simulink model "X_to_ADD_fix"  (Simulink 7.0)
settings: Solver=FixedStepDiscrete  SolverMode=SingleTasking  StartTime=0.0  StopTime=1100  FixedStep=Ts  RelTol=1e-3
values from neighbouring files (symbols this model uses):
  Ts = 1    [x_to_add_fix_init.m]
  x_data_nb = 16    [x_to_add_fix_init.m]
  x_range_nb = 16    [x_to_add_fix_init.m]
undefined symbols (not defined in the file or in its folder): xlipgetpartsetting
libraries: xbsIndex_r4 x55
settings Model: Creator=jboulet  LastModifiedBy=jboulet

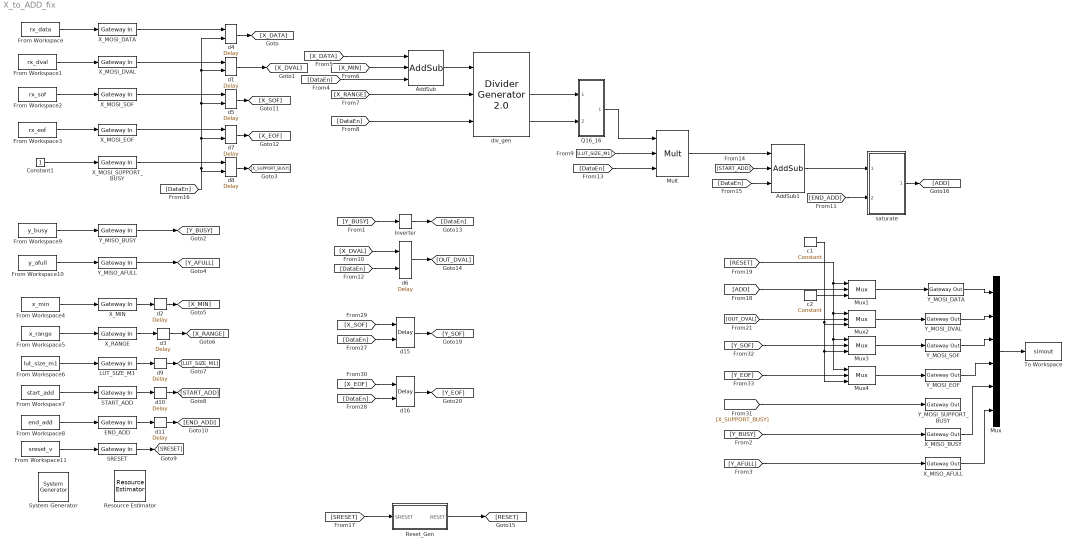
== system X_to_ADD_fix ==
  " System Generator" : xbsIndex_r4/ System Generator  Tag=genX  SystemSampleTime=-1  xilinxfamily=virtex4  part=xc4vfx100  speed=-10  package=ff1517  synthesis_tool=XST  clock_wrapper=Expose Clock Ports  directory=./ngc_netlist  testbench=off  simulink_period=1  sysclk_period=7.5  dcm_input_clock_period=100  incr_netlist=off  trim_vbits=Everywhere in SubSystem  dbl_ovrd=According to Block Masks  core_generation=According to Block Masks  run_coregen=off  deprecated_control=off  eval_field=0  block_type=sysgen
      settings: block_version=10.1.3
  AddSub : xbsIndex_r4/AddSub  mode=Subtraction  use_carryin=off  use_carryout=off  en=on  latency=1  precision=User Defined  arith_type=Unsigned  n_bits=16  bin_pt=0  quantization=Truncate  overflow=Saturate  dbl_ovrd=off  use_behavioral_HDL=off  pipelined=off  use_rpm=off  hw_selection=Fabric  block_type=addsub
      settings: xl_area=[8 16 0 16 0 0 0]  block_version=10.1.3
  AddSub1 : xbsIndex_r4/AddSub  mode=Addition  use_carryin=off  use_carryout=off  en=on  latency=1  precision=User Defined  arith_type=Unsigned  n_bits=end_add_nb  bin_pt=0  quantization=Truncate  overflow=Wrap  dbl_ovrd=off  use_behavioral_HDL=off  pipelined=off  use_rpm=on  hw_selection=Fabric  block_type=addsub
      settings: xl_area=[5 10 0 10 0 0 0]  block_version=10.1.3
  Constant1 : Constant
  END_ADD : xbsIndex_r4/Gateway In  arith_type=Unsigned  n_bits=end_add_nb  bin_pt=0  quantization=Truncate  overflow=Wrap  period=Ts  dbl_ovrd=off  timing_constraint=None  locs_specified=off  LOCs={}  block_type=gatewayin
      settings: infoedit="Gateway in block.  Converts inputs of type Simulink integer, double and fixed point to  Xilinx fixed point type.<P><P>Hardware notes:  In hardware these blocks become top level input ports."  xl_area=[0 0 0 0 10 0 0]  block_version=10.1.3
  From Workspace : FromWorkspace  VariableName=rx_data  SampleTime=Ts  Interpolate=off  OutputAfterFinalValue=Holding final value
  From Workspace1 : FromWorkspace  VariableName=rx_dval  SampleTime=Ts  Interpolate=off  OutputAfterFinalValue=Setting to zero
  From Workspace10 : FromWorkspace  VariableName=y_afull  SampleTime=Ts  Interpolate=off  OutputAfterFinalValue=Holding final value
  From Workspace11 : FromWorkspace  VariableName=sreset_v  SampleTime=Ts  Interpolate=off  OutputAfterFinalValue=Holding final value
  From Workspace2 : FromWorkspace  VariableName=rx_sof  SampleTime=Ts  Interpolate=off  OutputAfterFinalValue=Holding final value
  From Workspace3 : FromWorkspace  VariableName=rx_eof  SampleTime=Ts  Interpolate=off  OutputAfterFinalValue=Holding final value
  From Workspace4 : FromWorkspace  VariableName=x_min  SampleTime=Ts  Interpolate=off  OutputAfterFinalValue=Holding final value
  From Workspace5 : FromWorkspace  VariableName=x_range  SampleTime=Ts  Interpolate=off  OutputAfterFinalValue=Holding final value
  From Workspace6 : FromWorkspace  VariableName=lut_size_m1  SampleTime=Ts  Interpolate=off  OutputAfterFinalValue=Holding final value
  From Workspace7 : FromWorkspace  VariableName=start_add  SampleTime=Ts  Interpolate=off  OutputAfterFinalValue=Holding final value
  From Workspace8 : FromWorkspace  VariableName=end_add  SampleTime=Ts  Interpolate=off  OutputAfterFinalValue=Holding final value
  From Workspace9 : FromWorkspace  VariableName=y_busy  SampleTime=Ts  Interpolate=off  OutputAfterFinalValue=Holding final value
  Inverter : xbsIndex_r4/Inverter  en=off  latency=0  dbl_ovrd=off  block_type=inv
      settings: xl_area=[0 0 0 0 0 0 0]
  LUT_SIZE_M1 : xbsIndex_r4/Gateway In  arith_type=Unsigned  n_bits=lut_size_m1_nb  bin_pt=0  quantization=Truncate  overflow=Wrap  period=Ts  dbl_ovrd=off  timing_constraint=None  locs_specified=off  LOCs={}  block_type=gatewayin
      settings: infoedit="Gateway in block.  Converts inputs of type Simulink integer, double and fixed point to  Xilinx fixed point type.<P><P>Hardware notes:  In hardware these blocks become top level input ports."  xl_area=[0 0 0 0 10 0 0]  block_version=10.1.3
  Mult : xbsIndex_r4/Mult  precision=User Defined  arith_type=Unsigned  n_bits=end_add_nb  bin_pt=0  quantization=Truncate  overflow=Wrap  en=on  latency=3  dbl_ovrd=off  use_behavioral_HDL=off  use_embedded=off  opt=Speed  optimum_pipeline=off  pipeline=on  use_rpm=on  placement_style=Triangular  block_type=mult
      settings: infoedit=Hardware notes: To use the internal pipeline stage of the dedicated multiplier you must select 'Pipeline for maximum performance'.  xl_area=[119 209 0 198 0 0 0]  block_version=10.1.3
  Mux : Mux  Inputs=6
  Mux{1..4} (4 alike) : xbsIndex_r4/Mux  inputs=2  en=off  latency=0  precision=Full  arith_type=Unsigned  n_bits=16  bin_pt=14  quantization=Truncate  overflow=Wrap  dbl_ovrd=off  block_type=mux
  Q16_16 : Subsystem
  Reset_Gen : Subsystem
  Resource Estimator : xbsIndex_r4/Resource Estimator  Tag=resEstTag  Slices=88  FFs=61  BRAMs=1  LUTs=84  IOBs=48  EBMs=0  TBUFs=0  xl_use_estimator_area=off  est_options=Estimate  xl_estimator_area=[188 318 0 246 137 0 0]  block_type=resource_estimator
      settings: AttributesFormatString=Resource\nEstimator  block_version=10.1.3
  SRESET : xbsIndex_r4/Gateway In  arith_type=Boolean  n_bits=8  bin_pt=0  quantization="Round  (unbiased: +/- Inf)"  overflow=Wrap  period=1  dbl_ovrd=off  timing_constraint=None  locs_specified=off  LOCs={}  block_type=gatewayin
      settings: infoedit="Gateway in block.  Converts inputs of type Simulink integer, double and fixed point to  Xilinx fixed point type.<P><P>Hardware notes:  In hardware these blocks become top level input ports."  xl_area=[0 0 0 0 1 0 0]  block_version=10.1.3
  START_ADD : xbsIndex_r4/Gateway In  arith_type=Unsigned  n_bits=start_add_nb  bin_pt=0  quantization=Truncate  overflow=Wrap  period=Ts  dbl_ovrd=off  timing_constraint=None  locs_specified=off  LOCs={}  block_type=gatewayin
      settings: infoedit="Gateway in block.  Converts inputs of type Simulink integer, double and fixed point to  Xilinx fixed point type.<P><P>Hardware notes:  In hardware these blocks become top level input ports."  xl_area=[0 0 0 0 10 0 0]  block_version=10.1.3
  To Workspace : ToWorkspace  VariableName=simout  SampleTime=-1  SaveFormat=Structure
  X_MIN : xbsIndex_r4/Gateway In  arith_type=Unsigned  n_bits=x_min_nb  bin_pt=0  quantization=Truncate  overflow=Wrap  period=Ts  dbl_ovrd=off  timing_constraint=None  locs_specified=off  LOCs={}  block_type=gatewayin
      settings: infoedit="Gateway in block.  Converts inputs of type Simulink integer, double and fixed point to  Xilinx fixed point type.<P><P>Hardware notes:  In hardware these blocks become top level input ports."  xl_area=[0 0 0 0 16 0 0]  block_version=10.1.3
  X_MISO_AFULL : xbsIndex_r4/Gateway Out  hdl_port=on  timing_constraint=None  locs_specified=off  LOCs={}  block_type=gatewayout
      settings: infoedit="Gateway out block.  Converts Xilinx fixed point inputs into ouputs of type Simulink integer, double, or fixed point.<P><P>Hardware notes:  In hardware these blocks become top level output ports or are discarded, depending on how they are configured."  xl_area=[0 0 0 0 1 0 0]  block_version=10.1.3
  X_MISO_BUSY : xbsIndex_r4/Gateway Out  hdl_port=on  timing_constraint=None  locs_specified=off  LOCs={}  block_type=gatewayout
      settings: infoedit="Gateway out block.  Converts Xilinx fixed point inputs into ouputs of type Simulink integer, double, or fixed point.<P><P>Hardware notes:  In hardware these blocks become top level output ports or are discarded, depending on how they are configured."  xl_area=[0 0 0 0 1 0 0]  block_version=10.1.3
  X_MOSI_DATA : xbsIndex_r4/Gateway In  arith_type=Unsigned  n_bits=x_data_nb  bin_pt=0  quantization=Truncate  overflow=Wrap  period=Ts  dbl_ovrd=off  timing_constraint=None  locs_specified=off  LOCs={}  block_type=gatewayin
      settings: infoedit="Gateway in block.  Converts inputs of type Simulink integer, double and fixed point to  Xilinx fixed point type.<P><P>Hardware notes:  In hardware these blocks become top level input ports."  xl_area=[0 0 0 0 16 0 0]  block_version=10.1.3
  X_MOSI_DVAL : xbsIndex_r4/Gateway In  arith_type=Boolean  n_bits=8  bin_pt=0  quantization="Round  (unbiased: +/- Inf)"  overflow=Wrap  period=1  dbl_ovrd=off  timing_constraint=None  locs_specified=off  LOCs={}  block_type=gatewayin
      settings: infoedit="Gateway in block.  Converts inputs of type Simulink integer, double and fixed point to  Xilinx fixed point type.<P><P>Hardware notes:  In hardware these blocks become top level input ports."  xl_area=[0 0 0 0 1 0 0]  block_version=10.1.3
  X_MOSI_EOF : xbsIndex_r4/Gateway In  arith_type=Boolean  n_bits=8  bin_pt=0  quantization="Round  (unbiased: +/- Inf)"  overflow=Wrap  period=1  dbl_ovrd=off  timing_constraint=None  locs_specified=off  LOCs={}  block_type=gatewayin
      settings: infoedit="Gateway in block.  Converts inputs of type Simulink integer, double and fixed point to  Xilinx fixed point type.<P><P>Hardware notes:  In hardware these blocks become top level input ports."  xl_area=[0 0 0 0 1 0 0]  block_version=10.1.3
  X_MOSI_SOF : xbsIndex_r4/Gateway In  arith_type=Boolean  n_bits=8  bin_pt=0  quantization="Round  (unbiased: +/- Inf)"  overflow=Wrap  period=1  dbl_ovrd=off  timing_constraint=None  locs_specified=off  LOCs={}  block_type=gatewayin
      settings: infoedit="Gateway in block.  Converts inputs of type Simulink integer, double and fixed point to  Xilinx fixed point type.<P><P>Hardware notes:  In hardware these blocks become top level input ports."  xl_area=[0 0 0 0 1 0 0]  block_version=10.1.3
  X_MOSI_SUPPORT_BUSY : xbsIndex_r4/Gateway In  arith_type=Boolean  n_bits=8  bin_pt=0  quantization="Round  (unbiased: +/- Inf)"  overflow=Wrap  period=1  dbl_ovrd=off  timing_constraint=None  locs_specified=off  LOCs={}  block_type=gatewayin
      settings: infoedit="Gateway in block.  Converts inputs of type Simulink integer, double and fixed point to  Xilinx fixed point type.<P><P>Hardware notes:  In hardware these blocks become top level input ports."  xl_area=[0 0 0 0 1 0 0]  block_version=10.1.3
  X_RANGE : xbsIndex_r4/Gateway In  arith_type=Unsigned  n_bits=x_range_nb  bin_pt=0  quantization=Truncate  overflow=Wrap  period=Ts  dbl_ovrd=off  timing_constraint=None  locs_specified=off  LOCs={}  block_type=gatewayin
      settings: infoedit="Gateway in block.  Converts inputs of type Simulink integer, double and fixed point to  Xilinx fixed point type.<P><P>Hardware notes:  In hardware these blocks become top level input ports."  xl_area=[0 0 0 0 16 0 0]  block_version=10.1.3
  Y_MISO_AFULL : xbsIndex_r4/Gateway In  arith_type=Boolean  n_bits=8  bin_pt=0  quantization="Round  (unbiased: +/- Inf)"  overflow=Wrap  period=1  dbl_ovrd=off  timing_constraint=None  locs_specified=off  LOCs={}  block_type=gatewayin
      settings: infoedit="Gateway in block.  Converts inputs of type Simulink integer, double and fixed point to  Xilinx fixed point type.<P><P>Hardware notes:  In hardware these blocks become top level input ports."  xl_area=[0 0 0 0 1 0 0]  block_version=10.1.3
  Y_MISO_BUSY : xbsIndex_r4/Gateway In  arith_type=Boolean  n_bits=8  bin_pt=0  quantization="Round  (unbiased: +/- Inf)"  overflow=Wrap  period=1  dbl_ovrd=off  timing_constraint=None  locs_specified=off  LOCs={}  block_type=gatewayin
      settings: infoedit="Gateway in block.  Converts inputs of type Simulink integer, double and fixed point to  Xilinx fixed point type.<P><P>Hardware notes:  In hardware these blocks become top level input ports."  xl_area=[0 0 0 0 1 0 0]  block_version=10.1.3
  Y_MOSI_DATA : xbsIndex_r4/Gateway Out  hdl_port=on  timing_constraint=None  locs_specified=off  LOCs={}  block_type=gatewayout
      settings: infoedit="Gateway out block.  Converts Xilinx fixed point inputs into ouputs of type Simulink integer, double, or fixed point.<P><P>Hardware notes:  In hardware these blocks become top level output ports or are discarded, depending on how they are configured."  xl_area=[0 0 0 0 10 0 0]  block_version=10.1.3
  Y_MOSI_DVAL : xbsIndex_r4/Gateway Out  hdl_port=on  timing_constraint=None  locs_specified=off  LOCs={}  block_type=gatewayout
      settings: infoedit="Gateway out block.  Converts Xilinx fixed point inputs into ouputs of type Simulink integer, double, or fixed point.<P><P>Hardware notes:  In hardware these blocks become top level output ports or are discarded, depending on how they are configured."  xl_area=[0 0 0 0 10 0 0]  block_version=10.1.3
  Y_MOSI_EOF : xbsIndex_r4/Gateway Out  hdl_port=on  timing_constraint=None  locs_specified=off  LOCs={}  block_type=gatewayout
      settings: infoedit="Gateway out block.  Converts Xilinx fixed point inputs into ouputs of type Simulink integer, double, or fixed point.<P><P>Hardware notes:  In hardware these blocks become top level output ports or are discarded, depending on how they are configured."  xl_area=[0 0 0 0 10 0 0]  block_version=10.1.3
  Y_MOSI_SOF : xbsIndex_r4/Gateway Out  hdl_port=on  timing_constraint=None  locs_specified=off  LOCs={}  block_type=gatewayout
      settings: infoedit="Gateway out block.  Converts Xilinx fixed point inputs into ouputs of type Simulink integer, double, or fixed point.<P><P>Hardware notes:  In hardware these blocks become top level output ports or are discarded, depending on how they are configured."  xl_area=[0 0 0 0 10 0 0]  block_version=10.1.3
  Y_MOSI_SUPPORT_BUSY : xbsIndex_r4/Gateway Out  hdl_port=on  timing_constraint=None  locs_specified=off  LOCs={}  block_type=gatewayout
      settings: infoedit="Gateway out block.  Converts Xilinx fixed point inputs into ouputs of type Simulink integer, double, or fixed point.<P><P>Hardware notes:  In hardware these blocks become top level output ports or are discarded, depending on how they are configured."  xl_area=[0 0 0 0 10 0 0]  block_version=10.1.3
  c1 : xbsIndex_r4/Constant  arith_type=Boolean  const=0  n_bits=16  bin_pt=14  explicit_period=off  period=1  equ=P=C  opselect=C  inp2=PCIN>>17  opr=+  inp1=P  carry=CIN  dbl_ovrd=off  block_type=constant
  c2 : xbsIndex_r4/Constant  arith_type=Unsigned  const=0  n_bits=16  bin_pt=0  explicit_period=off  period=1  equ=P=C  opselect=C  inp2=PCIN>>17  opr=+  inp1=P  carry=CIN  dbl_ovrd=off  block_type=constant
  d{1,4..5,7..8} (5 alike) : xbsIndex_r4/Delay  en=on  latency=1  dbl_ovrd=off  reg_retiming=off  block_type=delay
      settings: xl_area=[8 16 0 0 0 0 0]
  d{2..3,9..11} (5 alike) : xbsIndex_r4/Delay  en=off  latency=1  dbl_ovrd=off  reg_retiming=off  block_type=delay
      d10 settings: xl_area=[5 10 0 0 0 0 0]
      d11 settings: xl_area=[5 10 0 0 0 0 0]
      d2 settings: xl_area=[8 16 0 0 0 0 0]
      d3 settings: xl_area=[8 16 0 0 0 0 0]
      d9 settings: xl_area=[5 10 0 0 0 0 0]
  d15 : xbsIndex_r4/Delay  en=on  latency=x_data_nb+x_range_nb+2+5  dbl_ovrd=off  reg_retiming=off  block_type=delay
      settings: xl_area=[1 1 0 0 0 0 0]
  d16 : xbsIndex_r4/Delay  en=on  latency=x_data_nb+x_range_nb+2+5  dbl_ovrd=off  reg_retiming=off  block_type=delay
      settings: xl_area=[1 1 0 0 0 0 0]
  d6 : xbsIndex_r4/Delay  en=on  latency=x_data_nb+x_range_nb+2+5  dbl_ovrd=off  reg_retiming=off  block_type=delay
      settings: xl_area=[1 1 0 0 0 0 0]
  div_gen : xbsIndex_r4/Divider Generator 2.0   dividend_and_quotient_width=x_data_nb  divisor_width=x_range_nb  algorithm_type=Radix2  remainder_type=Fractional  fractional_width=16  clocks_per_division=1  divide_by_zero_detect=off  latency_configuration=Automatic  latency=1  en=on  rst=off  ip_name=Divider Generator  ip_version=2.0  dsptool_ready=true  wrapper_available=true  ce=1  sclr=1  sclr_ce_priority=SCLR_overrides_CE  operand_sign=Signed  port_translation_map={ 'ce' => 'en', 'sclr' => 'rst' }  ipcore_fpga_part=xlipgetpartsetting(gcb, {'virtex4', 'xc4vsx35', '-10', 'ff668'})  block_type=div_gen_v2_0
      settings: block_version=10.1.3
  saturate : Subsystem
  wires:
  From Workspace1/1 -> X_MOSI_DVAL/1
  X_MOSI_DVAL/1 -> d1/1
  X_MOSI_DATA/1 -> d4/1
  From Workspace3/1 -> X_MOSI_EOF/1
  From Workspace2/1 -> X_MOSI_SOF/1
  X_MOSI_EOF/1 -> d7/1
  X_MOSI_SOF/1 -> d5/1
  From Workspace/1 -> X_MOSI_DATA/1
  From Workspace11/1 -> SRESET/1
  SRESET/1 -> [SRESET]
  X_MOSI_SUPPORT_BUSY/1 -> d8/1
  Constant1/1 -> X_MOSI_SUPPORT_BUSY/1
  X_MIN/1 -> d2/1
  From Workspace4/1 -> X_MIN/1
  From Workspace5/1 -> X_RANGE/1
  LUT_SIZE_M1/1 -> d9/1
  From Workspace6/1 -> LUT_SIZE_M1/1
  START_ADD/1 -> d10/1
  From Workspace7/1 -> START_ADD/1
  END_ADD/1 -> d11/1
  From Workspace8/1 -> END_ADD/1
  Y_MISO_BUSY/1 -> [Y_BUSY]
  Y_MISO_AFULL/1 -> [Y_AFULL]
  d4/1 -> [X_DATA]
  d1/1 -> [X_DVAL]
  d8/1 -> [X_SUPPORT_BUSY]
  d2/1 -> [X_MIN]
  d3/1 -> [X_RANGE]
  d9/1 -> [LUT_SIZE_M1]
  d10/1 -> [START_ADD]
  d11/1 -> [END_ADD]
  d5/1 -> [X_SOF]
  d7/1 -> [X_EOF]
  [X_DATA] -> AddSub/1
  [X_MIN] -> AddSub/2
  [DataEn] -> AddSub/3
  AddSub/1 -> div_gen/1
  [X_RANGE] -> div_gen/2
  [LUT_SIZE_M1] -> Mult/2
  Mult/1 -> AddSub1/1
  [START_ADD] -> AddSub1/2
  AddSub1/1 -> saturate/1(Add_IN)
  [END_ADD] -> saturate/2(end_add)
  [Y_BUSY] -> Inverter/1
  Inverter/1 -> [DataEn]
  X_RANGE/1 -> d3/1
  div_gen/2 -> Q16_16/1(In1)
  div_gen/3 -> Q16_16/2(In2)
  Q16_16/1(Out1) -> Mult/1
  [DataEn] -> Mult/3
  [DataEn] -> AddSub1/3
  [X_SOF] -> d15/1
  [DataEn] -> d15/2
  [X_EOF] -> d16/1
  [DataEn] -> d16/2
  d15/1 -> [Y_SOF]
  d16/1 -> [Y_EOF]
  [DataEn] -> div_gen/3
  Y_MOSI_DATA/1 -> Mux/1
  Y_MOSI_DVAL/1 -> Mux/2
  Y_MOSI_SOF/1 -> Mux/3
  Y_MOSI_EOF/1 -> Mux/4
  Mux/1 -> To Workspace/1
  From Workspace9/1 -> Y_MISO_BUSY/1
  From Workspace10/1 -> Y_MISO_AFULL/1
  [X_DVAL] -> d6/1
  d6/1 -> [OUT_DVAL]
  [DataEn] -> d6/2
  X_MISO_BUSY/1 -> Mux/5
  X_MISO_AFULL/1 -> Mux/6
  [DataEn] -> d4/2, d1/2, d5/2, d7/2, d8/2
  [SRESET] -> Reset_Gen/1(SRESET)
  Reset_Gen/1(RESET) -> [RESET]
  saturate/1(add_out) -> [ADD]
  Mux1/1 -> Y_MOSI_DATA/1
  [RESET] -> Mux1/1, Mux2/1, Mux3/1, Mux4/1
  [ADD] -> Mux1/2
  [OUT_DVAL] -> Mux2/2
  [Y_SOF] -> Mux3/2
  [Y_EOF] -> Mux4/2
  [X_SUPPORT_BUSY] -> Y_MOSI_SUPPORT_BUSY/1
  [Y_BUSY] -> X_MISO_BUSY/1
  [Y_AFULL] -> X_MISO_AFULL/1
  Mux2/1 -> Y_MOSI_DVAL/1
  Mux3/1 -> Y_MOSI_SOF/1
  Mux4/1 -> Y_MOSI_EOF/1
  c1/1 -> Mux2/3, Mux3/3, Mux4/3
  c2/1 -> Mux1/3

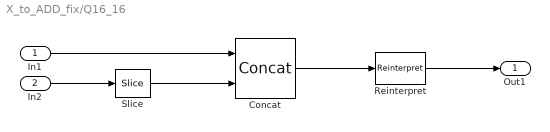
== system X_to_ADD_fix/Q16_16 ==
  In1 : Inport
  In2 : Inport  Port=2
  Concat : xbsIndex_r4/Concat  num_inputs=2  dbl_ovrd=off  block_type=concat
      settings: block_version=10.1.3
  Reinterpret : xbsIndex_r4/Reinterpret  force_arith_type=on  arith_type=Unsigned  force_bin_pt=on  bin_pt=x_range_nb  block_type=reinterpret
      settings: infoedit="Changes signal type without altering the binary representation.   You can changed the signal between signed and unsigned, and relocate the binary point.<P><P>Hardware notes: In hardware this block costs nothing.<P><P>Example:  Suppose the input is 6 bits wide, signed, with 2 fractional bits, and the output is forced to unsigned with 0 fractional bits.  Then an input of -2.0 (1110.00 in binary 2's complement) becomes an output of 56 (111000 in binary)."  block_version=10.1.3
  Slice : xbsIndex_r4/Slice  nbits=x_range_nb  boolean_output=off  mode=Lower Bit Location + Width  bit1=0  base1=LSB of Input  bit0=0  base0=LSB of Input  dbl_ovrd=off  block_type=slice
      settings: infoedit="Extracts a given range of bits from each input sample and presents it at the output.  The output type is ordinarily unsigned with binary point at zero, but can be Boolean when the slice is one bit wide.<P><P>Hardware notes: In hardware this block costs nothing."  block_version=10.1.3
  Out1 : Outport
  wires:
  In2/1 -> Slice/1
  In1/1 -> Concat/1
  Slice/1 -> Concat/2
  Concat/1 -> Reinterpret/1
  Reinterpret/1 -> Out1/1

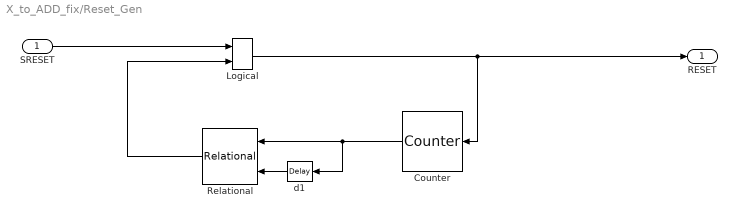
== system X_to_ADD_fix/Reset_Gen ==
  SRESET : Inport  OutDataType=sfix(16)  OutScaling=2^0
  Counter : xbsIndex_r4/Counter  Orientation=left  cnt_type=Count Limited  cnt_to=x_data_nb+x_range_nb+2+5+1  operation=Up  start_count=0  cnt_by_val=1  arith_type=Unsigned  n_bits=ceil(log2(x_data_nb+x_range_nb+2+5+1))  bin_pt=0  load_pin=off  rst=off  en=on  explicit_period=on  period=1  dbl_ovrd=off  use_behavioral_HDL=off  use_rpm=off  implementation=Fabric  block_type=counter
  Logical : xbsIndex_r4/Logical  logical_function=OR  inputs=2  en=off  latency=0  precision=Full  arith_type=Unsigned  n_bits=16  bin_pt=0  align_bp=on  dbl_ovrd=off  block_type=logical
  Relational : xbsIndex_r4/Relational  Orientation=left  mode=a>b  en=off  latency=0  dbl_ovrd=off  block_type=relational
      settings: block_version=10.1.3
  d1 : xbsIndex_r4/Delay  Orientation=left  en=off  latency=1  dbl_ovrd=off  reg_retiming=off  block_type=delay
  RESET : Outport  OutDataType=sfix(16)  OutScaling=2^0
  wires:
  d1/1 -> Relational/2
  SRESET/1 -> Logical/1
  Relational/1 -> Logical/2
  Counter/1 -> Relational/1, d1/1
  Logical/1 -> Counter/1, RESET/1

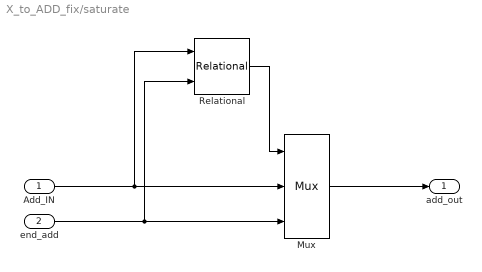
== system X_to_ADD_fix/saturate ==
  Add_IN : Inport  OutDataType=sfix(16)  OutScaling=2^0
  end_add : Inport  Port=2  OutDataType=sfix(16)  OutScaling=2^0
  Mux : xbsIndex_r4/Mux  inputs=2  en=off  latency=0  precision=User Defined  arith_type=Unsigned  n_bits=end_add_nb  bin_pt=0  quantization=Truncate  overflow=Wrap  dbl_ovrd=off  block_type=mux
      settings: xl_area=[5 0 0 10 0 0 0]
  Relational : xbsIndex_r4/Relational  mode=a>=b  en=off  latency=0  dbl_ovrd=off  block_type=relational
      settings: xl_area=[6 0 0 11 0 0 0]  block_version=10.1.3
  add_out : Outport  OutDataType=sfix(16)  OutScaling=2^0
  wires:
  Relational/1 -> Mux/1
  Add_IN/1 -> Mux/2, Relational/1
  end_add/1 -> Mux/3, Relational/2
  Mux/1 -> add_out/1
